simulink model "project_6"  (R2020a)
settings: Solver=VariableStepAuto  StartTime=0.0  StopTime=10.0  MaxStep=0.01  RelTol=1e-3
values from neighbouring files (symbols this model uses):
  Kd = 50    [project_7m.m]    (also in project_8m.m = 207.6; project_9m.m = 2)
  Ki = 300    [project_7m.m]    (also in project_8m.m = 7398; project_9m.m = 4)
  Kp = 1    [project_6m.m]    (also in project_7m.m = 350; project_8m.m = 4433; project_9m.m = 8000)
settings Model: Creator=Matt  LastModifiedBy=Matt
settings DataIOCC: ReturnWorkspaceOutputs=off  TimeSaveName=time

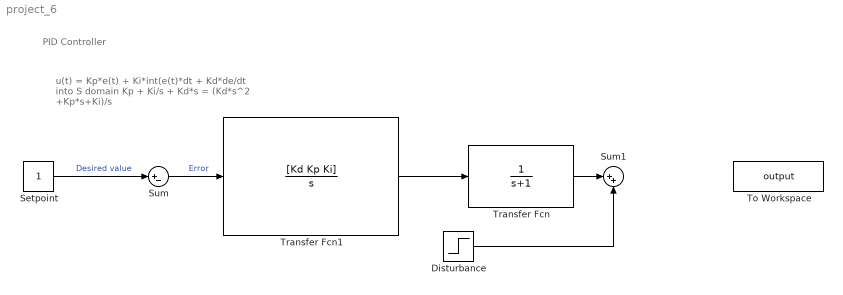
== system project_6 ==
  note: u(t) = Kp*e(t) + Ki*int(e(t)*dt + Kd*de/dt
      | into S domain
      | Kp + Ki/s + Kd*s = (Kd*s^2 +Kp*s+Ki)/s
  note: PID Controller
  Disturbance : Step  SampleTime=0
  Setpoint : Constant
  Sum : Sum  Inputs=|+-
  Sum1 : Sum  Inputs=|++
  To Workspace : ToWorkspace  VariableName=output  SampleTime=-1
  Transfer Fcn : TransferFcn  Denominator=[1 1]
  Transfer Fcn1 : TransferFcn  Numerator=[Kd Kp Ki]  Denominator=[1 0]
  wires:
  Setpoint/1 -> Sum/1  "Desired value"
  Sum/1 -> Transfer Fcn1/1  "Error"
  Transfer Fcn1/1 -> Transfer Fcn/1
  Transfer Fcn/1 -> Sum1/1
  Disturbance/1 -> Sum1/2
  ? -> To Workspace/1
